simulink model "PIDcontroller"  (R2024b)
settings: Solver=VariableStepAuto  StartTime=0.0  StopTime=10.0  RelTol=1e-3
values from neighbouring files (symbols this model uses):
  Ki = chro(2)    [RGA_fitfun.m]    (also in RGA_main.m = minimum_Kp_Ki_Kd(2))
  Kp = chro(1)    [RGA_fitfun.m]    (also in RGA_main.m = minimum_Kp_Ki_Kd(1))
  target_value = target_value + (1 + 2*rand)    [RGA_main.m]
settings Model: Creator=User  LastModifiedBy=Pin Chuen
settings SolverCC: AlgebraicLoopSolver=LineSearch
settings DebuggingCC: AlgebraicLoopMsg=none  UnconnectedInputMsg=warning  UnconnectedOutputMsg=warning  UnconnectedLineMsg=warning
settings ModelReferenceCC: EnableRefExpFcnMdlSchedulingChecks=on
settings SFSimCC: CustomCodeUndefinedFunction=UseInterfaceOnly
settings RTWCC: GPUComputeCapability=3.5

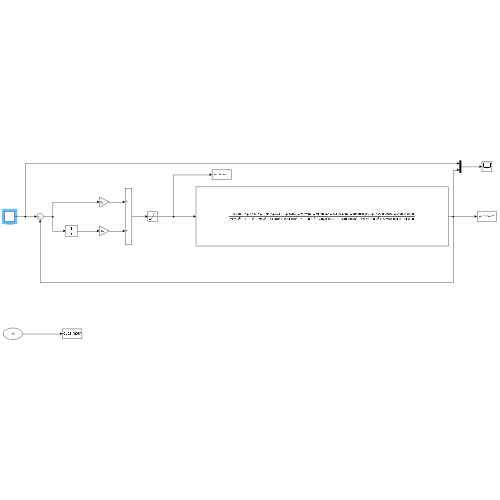
[thumbnail: Simulink's stored preview of the top-level diagram]
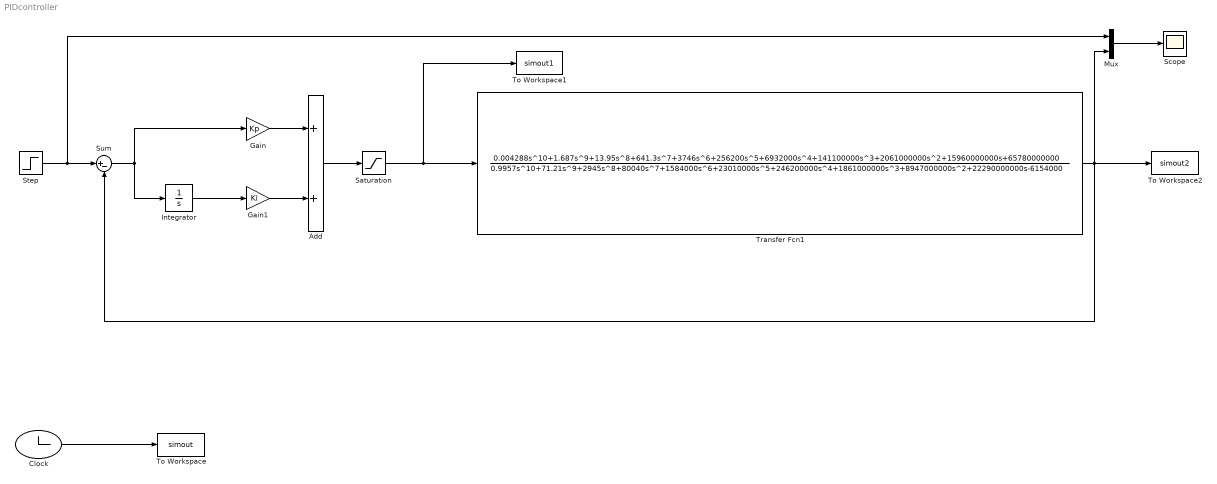
== system PIDcontroller ==
  Add : Sum
  Clock : Clock
  Gain : Gain  Gain=Kp
  Gain1 : Gain  Gain=Ki
  Integrator : Integrator
  Mux : Mux  Inputs=2
  Saturation : Saturate  UpperLimit=60  LowerLimit=-60
  Scope : Scope
  Step : Step  Before=target_value  After=target_value  SampleTime=0
  Sum : Sum  Inputs=|+-
  To Workspace : ToWorkspace  VariableName=simout  SampleTime=-1
      settings: Save2DSignal=2-D array (concatenate along first dimension)
  To Workspace1 : ToWorkspace  VariableName=simout1  SampleTime=-1
      settings: Save2DSignal=2-D array (concatenate along first dimension)
  To Workspace2 : ToWorkspace  VariableName=simout2  SampleTime=-1
      settings: Save2DSignal=2-D array (concatenate along first dimension)
  Transfer Fcn1 : TransferFcn  Numerator=[0.004288 1.687 13.95 641.3 3746 256200 6932000 141100000 2061000000 15960000000 65780000000]  Denominator=[0.9957 71.21 2945 80040 1584000 23010000 246200000 1861000000 8947000000 22290000000 -6154000]
  wires:
  Gain/1 -> Add/1
  Gain1/1 -> Add/2
  Integrator/1 -> Gain1/1
  Sum/1 -> Gain/1, Integrator/1
  Step/1 -> Mux/1, Sum/1
  Clock/1 -> To Workspace/1
  Mux/1 -> Scope/1
  Add/1 -> Saturation/1
  Transfer Fcn1/1 -> Sum/2, Mux/2, To Workspace2/1
  Saturation/1 -> Transfer Fcn1/1, To Workspace1/1
